simulink model "sistemaConsignadeTorque"  (R2017a)
settings: Solver=ode45  StartTime=0.0  StopTime=10.0  RelTol=1e-3  EnableMultiTasking=on
values from neighbouring files (symbols this model uses):
  alfa_cu = 3.9*10^-3    (= 0.0039)    [InicializaYconstantes.m]
  b_m = bm+(bl/r^2)    (= 1.5e-05)    [InicializaYconstantes.m]
  Cts = 1.091    [InicializaYconstantes.m]
  J_m = Jm+(Jl/r^2)    (= 5.65099476805e-06)    [InicializaYconstantes.m]
  lambda = 0.01546    [InicializaYconstantes.m]
  Ld = 6.6*10^-3    (= 0.0066)    [InicializaYconstantes.m]
  Lq = 5.8*10^-3    (= 0.0058)    [InicializaYconstantes.m]
  Pp = 3    [InicializaYconstantes.m]
  R1 = -p1i*Lq    (= 29)    [InicializaYconstantes.m]
  R2 = -p1i*Ld    (= 33)    [InicializaYconstantes.m]
  Rs = 1.02    [InicializaYconstantes.m]
  Rs_cero = 1.02    [InicializaYconstantes.m]
  Rts = 55    [InicializaYconstantes.m]
  Ta = 40    [InicializaYconstantes.m]
settings Model: Creator=usuario  LastModifiedBy=usuario
settings DataIOCC: LimitDataPoints=on  SaveFormat=Array
settings OptimizationCC: ExpressionDepthLimit=2147483647  LifeSpan=inf
settings DebuggingCC: UnderspecifiedInitializationDetection=Classic  MergeDetectMultiDrivingBlocksExec=none  SolverPrmCheckMsg=warning  StateNameClashWarn=warning  SFUnexpectedBacktrackingDiag=warning  SFNoUnconditionalDefaultTransitionDiag=warning  SFExecutionAtInitializationDiag=none
settings HardwareCC: ProdBitPerPointer=32  ProdBitPerSizeT=32  ProdBitPerPtrDiffT=32  ProdLargestAtomicFloat=None  ProdIntDivRoundTo=Undefined  ProdEndianess=Unspecified  ProdWordSize=32  ProdHWDeviceType=32-bit Generic
settings ModelReferenceCC: PropagateSignalLabelsOutOfModel=off
settings GRTTargetCC: TargetLangStandard=C89/C90 (ANSI)  GeneratePreprocessorConditionals=Disable all
settings ConfigComp: CovMetricSettings=dw  CovHtmlReporting=on  CovSaveCumulativeToWorkspaceVar=on  CovSaveSingleToWorkspaceVar=on  CovExternalEMLEnable=off

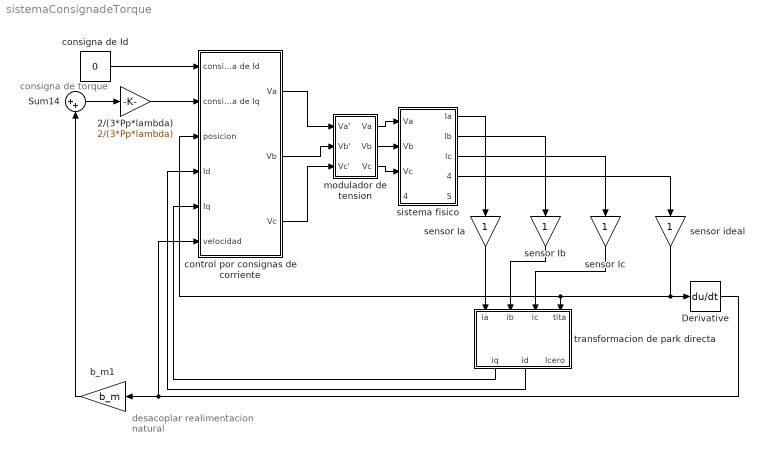
== system sistemaConsignadeTorque ==
  note: consigna
      | de torque
  note: desacoplar
      | realimentacion natural
  2/(3*Pp*lambda) : Gain  Gain=2/(3*Pp*lambda)
  Derivative : Derivative
  Sum14 : Sum  Inputs=|++
  b_m1 : Gain  Gain=b_m
  consigna de Id : Constant  Value=0
  control por consignas de corriente : Subsystem
  modulador de tension : Subsystem
  sensor Ia : Gain
  sensor Ib : Gain
  sensor Ic : Gain
  sensor ideal : Gain
  sistema fisico : Subsystem
  transformacion de park directa : Subsystem
  wires:
  sensor Ia/1 -> transformacion de park directa/1(ia)
  sensor Ib/1 -> transformacion de park directa/2(ib)
  sensor Ic/1 -> transformacion de park directa/3(ic)
  consigna de Id/1 -> control por consignas de corriente/1(consigna de Id)
  2/(3*Pp*lambda)/1 -> control por consignas de corriente/2(consigna de Iq)
  Sum14/1 -> 2/(3*Pp*lambda)/1
  ? -> Sum14/1
  control por consignas de corriente/1(Va) -> modulador de tension/1(Va')
  control por consignas de corriente/2(Vb) -> modulador de tension/2(Vb')
  control por consignas de corriente/3(Vc) -> modulador de tension/3(Vc')
  modulador de tension/1(Va) -> sistema fisico/1(Va)
  modulador de tension/2(Vb) -> sistema fisico/2(Vb)
  modulador de tension/3(Vc) -> sistema fisico/3(Vc)
  sistema fisico/1(Ia) -> sensor Ia/1
  sistema fisico/2(Ib) -> sensor Ib/1
  sistema fisico/3(Ic) -> sensor Ic/1
  sistema fisico/4(posicion1) -> sensor ideal/1
  sensor ideal/1 -> control por consignas de corriente/3(posicion), transformacion de park directa/4(tita), Derivative/1
  Derivative/1 -> control por consignas de corriente/6(velocidad), b_m1/1
  b_m1/1 -> Sum14/2
  transformacion de park directa/2(id) -> control por consignas de corriente/4(Id)
  transformacion de park directa/1(iq) -> control por consignas de corriente/5(Iq)

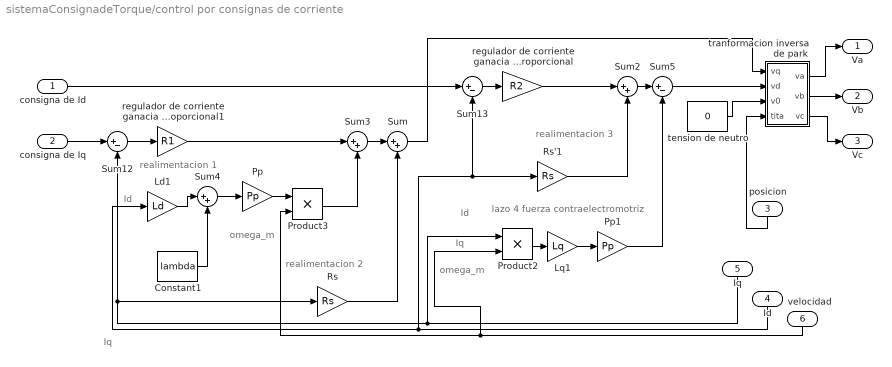
== system sistemaConsignadeTorque/control por consignas de corriente ==
  note: Id
  note: realimentacion 3
  note: Iq
  note: realimentacion 1
  note: Id
  note: omega_m
  note: realimentacion 2
  note: lazo 4 fuerza contraelectromotriz
  note: omega_m
  note: Iq
  consigna de Id : Inport
  consigna de Iq : Inport  Port=2
  posicion : Inport  Port=3
  Id : Inport  Port=4
  Iq : Inport  Port=5
  velocidad : Inport  Port=6
  Constant1 : Constant  Value=lambda
  Ld1 : Gain  Gain=Ld
  Lq1 : Gain  Gain=Lq
  Pp : Gain  Gain=Pp
  Pp1 : Gain  Gain=Pp
  Product2 : Product  RndMeth=Zero
  Product3 : Product  RndMeth=Zero
  Rs : Gain  Gain=Rs
  Rs'1 : Gain  Gain=Rs
  Sum{,2..4} (4 alike) : Sum  Inputs=|++
  Sum12 : Sum  Inputs=|+-
  Sum13 : Sum  Inputs=|+-
  Sum5 : Sum  Inputs=|+-
  regulador de corriente ganacia proporcional : Gain  Gain=R2
  regulador de corriente ganacia proporcional1 : Gain  Gain=R1
  tension de neutro : Constant  Value=0
  tranformacion inversa de park : Subsystem
  Va : Outport
  Vb : Outport  Port=2
  Vc : Outport  Port=3
  wires:
  regulador de corriente ganacia proporcional1/1 -> Sum3/1
  tension de neutro/1 -> tranformacion inversa de park/3(v0)
  Rs/1 -> Sum/2
  Sum4/1 -> Pp/1
  Constant1/1 -> Sum4/2
  Sum12/1 -> regulador de corriente ganacia proporcional1/1
  Sum5/1 -> tranformacion inversa de park/2(vd)
  tranformacion inversa de park/1(va) -> Va/1
  tranformacion inversa de park/3(vc) -> Vc/1
  Ld1/1 -> Sum4/1
  Sum/1 -> tranformacion inversa de park/1(vq)
  Id/1 -> Ld1/1, Sum13/2, Rs'1/1
  Pp/1 -> Product3/1
  regulador de corriente ganacia proporcional/1 -> Sum2/1
  consigna de Id/1 -> Sum13/1
  Rs'1/1 -> Sum2/2
  consigna de Iq/1 -> Sum12/1
  tranformacion inversa de park/2(vb) -> Vb/1
  Sum13/1 -> regulador de corriente ganacia proporcional/1
  Product3/1 -> Sum3/2
  Sum3/1 -> Sum/1
  posicion/1 -> tranformacion inversa de park/4(tita)
  Product2/1 -> Lq1/1
  Iq/1 -> Product2/1, Sum12/2, Rs/1
  Lq1/1 -> Pp1/1
  Pp1/1 -> Sum5/2
  velocidad/1 -> Product3/2, Product2/2
  Sum2/1 -> Sum5/1

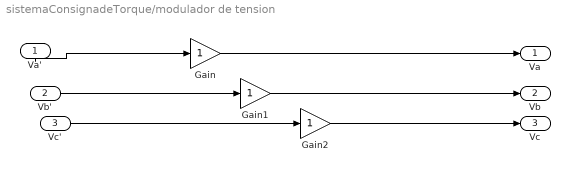
== system sistemaConsignadeTorque/modulador de tension ==
  Va' : Inport
  Vb' : Inport  Port=2
  Vc' : Inport  Port=3
  Gain : Gain
  Gain1 : Gain
  Gain2 : Gain
  Va : Outport
  Vb : Outport  Port=2
  Vc : Outport  Port=3
  wires:
  Gain/1 -> Va/1
  Gain1/1 -> Vb/1
  Vb'/1 -> Gain1/1
  Va'/1 -> Gain/1
  Vc'/1 -> Gain2/1
  Gain2/1 -> Vc/1

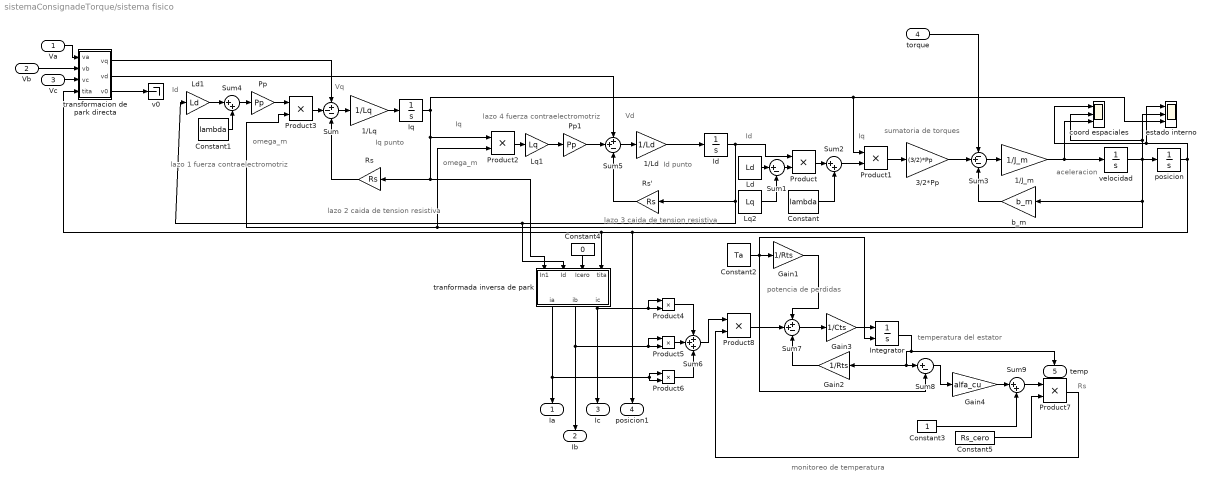
== system sistemaConsignadeTorque/sistema fisico ==
  note: potencia
      | de perdidas
  note: Rs
  note: lazo 4 fuerza contraelectromotriz
  note: lazo 3 caida de tension resistiva
  note: lazo 2 caida de tension resistiva
  note: lazo 1 fuerza contraelectromotriz
  note: sumatoria de torques
  note: Vd
  note: omega_m
  note: Iq
  note: Id punto
  note: Vq
  note: Id
  note: Iq punto
  note: Iq
  note: aceleracion
  note: Id
  note: omega_m
  note: monitoreo de temperatura
  note: temperatura del estator
  Va : Inport
  Vb : Inport  Port=2
  Vc : Inport  Port=3
  torque : Inport  Port=4
  1/J_m : Gain  Gain=1/J_m
  1/Ld : Gain  Gain=1/Ld
  1/Lq : Gain  Gain=1/Lq
  3/2*Pp : Gain  Gain=(3/2)*Pp
  Constant : Constant  Value=lambda
  Constant1 : Constant  Value=lambda
  Constant2 : Constant  Value=Ta
  Constant3 : Constant
  Constant4 : Constant  Value=0
  Constant5 : Constant  Value=Rs_cero
  Gain1 : Gain  Gain=1/Rts
  Gain2 : Gain  Gain=1/Rts
  Gain3 : Gain  Gain=1/Cts
  Gain4 : Gain  Gain=alfa_cu
  Id : Integrator
  Integrator : Integrator  InitialConditionSource=external
  Iq : Integrator
  Ld : Constant  Value=Ld
  Ld1 : Gain  Gain=Ld
  Lq1 : Gain  Gain=Lq
  Lq2 : Constant  Value=Lq
  Pp : Gain  Gain=Pp
  Pp1 : Gain  Gain=Pp
  Product{,1..8} (9 alike) : Product  RndMeth=Zero
  Rs : Gain  Gain=Rs
  Rs' : Gain  Gain=Rs
  Sum : Sum  Inputs=+--
  Sum1 : Sum  Inputs=|+-
  Sum2 : Sum  Inputs=|++
  Sum3 : Sum  Inputs=-+-
  Sum4 : Sum  Inputs=|++
  Sum5 : Sum  Inputs=++-
  Sum6 : Sum  Inputs=+++
  Sum7 : Sum  Inputs=++-
  Sum8 : Sum  Inputs=|+-
  Sum9 : Sum  Inputs=|++
  b_m : Gain  Gain=b_m
  coord espaciales : Scope  NumInputPorts=3
  estado interno : Scope  NumInputPorts=3
  posicion : Integrator
  "tranformada inversa de park " : Subsystem
  transformacion de park directa : Subsystem
  v0 : Terminator
  velocidad : Integrator  ContinuousStateAttributes='velocidad'
  Ia : Outport
  Ib : Outport  Port=2
  Ic : Outport  Port=3
  posicion1 : Outport  Port=4
  temp : Outport  Port=5
  wires:
  Product/1 -> Sum2/1
  Ld/1 -> Sum1/1
  Lq2/1 -> Sum1/2
  Sum1/1 -> Product/2
  Constant/1 -> Sum2/2
  Sum2/1 -> Product1/2
  1/Lq/1 -> Iq/1
  Product1/1 -> 3/2*Pp/1
  Ld1/1 -> Sum4/1
  Sum3/1 -> 1/J_m/1
  1/Ld/1 -> Id/1
  Constant1/1 -> Sum4/2
  b_m/1 -> Sum3/3
  Sum4/1 -> Pp/1
  Sum/1 -> 1/Lq/1
  Rs/1 -> Sum/3
  torque/1 -> Sum3/1
  Rs'/1 -> Sum5/3
  Product2/1 -> Lq1/1
  Iq/1 -> "tranformada inversa de park "/1(In1), Rs/1, Product2/1, estado interno/3, Product1/1
  Lq1/1 -> Pp1/1
  Product3/1 -> Sum/2
  transformacion de park directa/1(vq) -> Sum/1
  transformacion de park directa/2(vd) -> Sum5/1
  Sum5/1 -> 1/Ld/1
  3/2*Pp/1 -> Sum3/2
  1/J_m/1 -> velocidad/1, coord espaciales/3
  Pp1/1 -> Sum5/2
  transformacion de park directa/3(v0) -> v0/1
  posicion/1 -> coord espaciales/1, estado interno/1, transformacion de park directa/4(tita), "tranformada inversa de park "/4(tita), posicion1/1
  velocidad/1 -> posicion/1, Product3/2, Product2/2, b_m/1, estado interno/2, coord espaciales/2
  Pp/1 -> Product3/1
  Id/1 -> Rs'/1, Ld1/1, "tranformada inversa de park "/2(Id), Product/1
  Constant4/1 -> "tranformada inversa de park "/3(Icero)
  Vc/1 -> transformacion de park directa/3(vc)
  Vb/1 -> transformacion de park directa/2(vb)
  Va/1 -> transformacion de park directa/1(va)
  "tranformada inversa de park "/1(ia) -> Ia/1, Product6/2, Product6/1
  "tranformada inversa de park "/2(ib) -> Ib/1, Product5/1, Product5/2
  "tranformada inversa de park "/3(ic) -> Ic/1, Product4/1, Product4/2
  Product4/1 -> Sum6/1
  Product5/1 -> Sum6/2
  Product6/1 -> Sum6/3
  Product8/1 -> Sum7/2
  Constant2/1 -> Sum8/2, Gain1/1, Integrator/2
  Gain1/1 -> Sum7/1
  Sum7/1 -> Gain3/1
  Gain3/1 -> Integrator/1
  Integrator/1 -> temp/1, Sum8/1, Gain2/1
  Gain2/1 -> Sum7/3
  Sum8/1 -> Gain4/1
  Gain4/1 -> Sum9/1
  Constant3/1 -> Sum9/2
  Sum9/1 -> Product7/1
  Constant5/1 -> Product7/2
  Product7/1 -> Product8/2
  Sum6/1 -> Product8/1

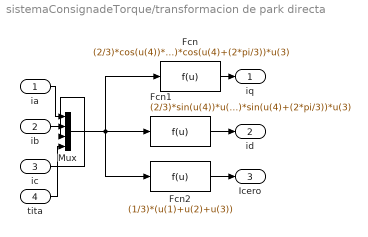
== system sistemaConsignadeTorque/transformacion de park directa ==
  ia : Inport
  ib : Inport  Port=2
  ic : Inport  Port=3
  tita : Inport  Port=4
  Fcn : Fcn  Expr=(2/3)*cos(u(4))*u(1)+(2/3)*cos(u(4)-(2*pi/3))*u(2)+(2/3)*cos(u(4)+(2*pi/3))*u(3)
  Fcn1 : Fcn  Expr=(2/3)*sin(u(4))*u(1)+(2/3)*sin(u(4)-(2*pi/3))*u(2)+(2/3)*sin(u(4)+(2*pi/3))*u(3)
  Fcn2 : Fcn  Expr=(1/3)*(u(1)+u(2)+u(3))
  Mux : Mux
  iq : Outport
  id : Outport  Port=2
  Icero : Outport  Port=3
  wires:
  Mux/1 -> Fcn1/1, Fcn/1, Fcn2/1
  Fcn/1 -> iq/1
  ia/1 -> Mux/1
  ib/1 -> Mux/2
  Fcn1/1 -> id/1
  ic/1 -> Mux/3
  tita/1 -> Mux/4
  Fcn2/1 -> Icero/1

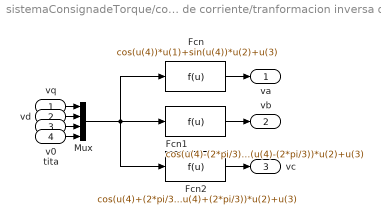
== system sistemaConsignadeTorque/control por consignas de corriente/tranformacion inversa de park ==
  vq : Inport
  vd : Inport  Port=2
  v0 : Inport  Port=3
  tita : Inport  Port=4
  Fcn : Fcn  Expr=cos(u(4))*u(1)+sin(u(4))*u(2)+u(3)
  Fcn1 : Fcn  Expr=cos(u(4)-(2*pi/3))*u(1)+sin(u(4)-(2*pi/3))*u(2)+u(3)
  Fcn2 : Fcn  Expr=cos(u(4)+(2*pi/3))*u(1)+sin(u(4)+(2*pi/3))*u(2)+u(3)
  Mux : Mux
  va : Outport
  vb : Outport  Port=2
  vc : Outport  Port=3
  wires:
  Mux/1 -> Fcn1/1, Fcn/1, Fcn2/1
  Fcn/1 -> va/1
  vq/1 -> Mux/1
  vd/1 -> Mux/2
  Fcn1/1 -> vb/1
  v0/1 -> Mux/3
  tita/1 -> Mux/4
  Fcn2/1 -> vc/1

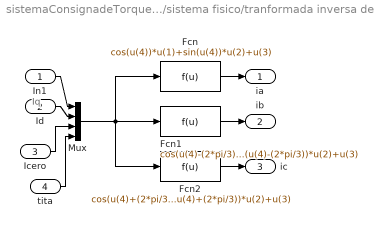
== system sistemaConsignadeTorque/sistema fisico/tranformada inversa de park  ==
  note: Iq
  In1 : Inport
  Id : Inport  Port=2
  Icero : Inport  Port=3
  tita : Inport  Port=4
  Fcn : Fcn  Expr=cos(u(4))*u(1)+sin(u(4))*u(2)+u(3)
  Fcn1 : Fcn  Expr=cos(u(4)-(2*pi/3))*u(1)+sin(u(4)-(2*pi/3))*u(2)+u(3)
  Fcn2 : Fcn  Expr=cos(u(4)+(2*pi/3))*u(1)+sin(u(4)+(2*pi/3))*u(2)+u(3)
  Mux : Mux
  ia : Outport
  ib : Outport  Port=2
  ic : Outport  Port=3
  wires:
  Mux/1 -> Fcn1/1, Fcn/1, Fcn2/1
  Fcn/1 -> ia/1
  In1/1 -> Mux/1
  Id/1 -> Mux/2
  Fcn1/1 -> ib/1
  Icero/1 -> Mux/3
  tita/1 -> Mux/4
  Fcn2/1 -> ic/1

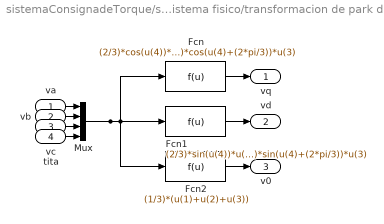
== system sistemaConsignadeTorque/sistema fisico/transformacion de park directa ==
  va : Inport
  vb : Inport  Port=2
  vc : Inport  Port=3
  tita : Inport  Port=4
  Fcn : Fcn  Expr=(2/3)*cos(u(4))*u(1)+(2/3)*cos(u(4)-(2*pi/3))*u(2)+(2/3)*cos(u(4)+(2*pi/3))*u(3)
  Fcn1 : Fcn  Expr=(2/3)*sin(u(4))*u(1)+(2/3)*sin(u(4)-(2*pi/3))*u(2)+(2/3)*sin(u(4)+(2*pi/3))*u(3)
  Fcn2 : Fcn  Expr=(1/3)*(u(1)+u(2)+u(3))
  Mux : Mux
  vq : Outport
  vd : Outport  Port=2
  v0 : Outport  Port=3
  wires:
  Mux/1 -> Fcn1/1, Fcn/1, Fcn2/1
  Fcn/1 -> vq/1
  va/1 -> Mux/1
  vb/1 -> Mux/2
  Fcn1/1 -> vd/1
  vc/1 -> Mux/3
  tita/1 -> Mux/4
  Fcn2/1 -> v0/1
